simulink model "kfs_pr_2"  (R2019a)
settings: Solver=FixedStepAuto  StartTime=0.0  StopTime=30000  FixedStep=1  RelTol=1e-3
values from neighbouring files (symbols this model uses):
  mb = 10800    [params.m]
  min_paus = 100    [params.m]
  nurk = deg2rad(0)    [params.m]
  vx_0 = 0    [params.m]
  vy_0 = 0    [params.m]
  x_0 = 0    [params.m]
  x_OK = 100    [params.m]
  y_0 = 0    [params.m]
  y_OK = 0    [params.m]
libraries: simulink_extras x4, simulink x3, dspswit3 x2
settings Model: Creator=Kasutaja  LastModifiedBy=Kasutaja
settings DataIOCC: ReturnWorkspaceOutputs=off
settings DebuggingCC: ArithmeticOperatorsInVariantConditions=warning

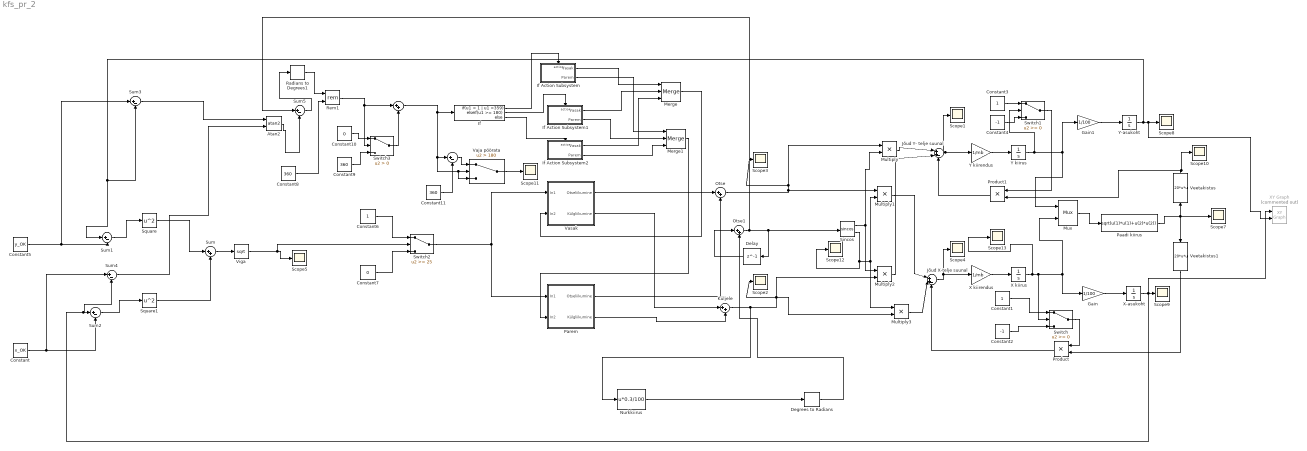
== system kfs_pr_2 ==
  " " : Sum  Inputs=|+-
  " " : Sum  Inputs=|++
  Atan2 : Trigonometry  Operator=atan2
  Constant : Constant  Value=x_OK
  Constant1 : Constant
  Constant10 : Constant  Value=0
  Constant11 : Constant  Value=360
  Constant2 : Constant  Value=-1
  Constant3 : Constant
  Constant4 : Constant  Value=-1
  Constant5 : Constant  Value=y_OK
  Constant6 : Constant
  Constant7 : Constant  Value=0
  Constant8 : Constant  Value=360
  Constant9 : Constant  Value=360
  Degrees to Radians : simulink_extras/Transformations/Degrees to Radians
  Delay : Delay  DelayLength=1  InitialCondition=nurk
  Gain : Gain  Gain=1/100
  Gain1 : Gain  Gain=1/100
  If : If  IfExpression=u1 < 1 | u1 >359  ElseIfExpressions=u1 >= 180
  If Action Subsystem : Subsystem  TreatAsAtomicUnit=on
  If Action Subsystem1 : Subsystem  TreatAsAtomicUnit=on
  If Action Subsystem2 : Subsystem  TreatAsAtomicUnit=on
  Jõud X-telje suunal : Sum  Inputs=|++-
  Jõud Y- telje suunal : Sum  Inputs=|++-
  Küljele : Sum  Inputs=|++
  Merge : Merge  Inputs=3
  Merge1 : Merge  Inputs=3
  Multiply{,1..3} (4 alike) : Product
  Mux : Mux  Inputs=2
      settings: DisplayOption=signals
  Nurkkiirus : Fcn  Expr=u*0.3/100
  Otse : Sum  Inputs=|++
  Otse1 : Sum  Inputs=|++
  Paadi kiirus : Fcn  Expr=sqrt(u(1)*u(1)+u(2)*u(2))
  Parem : Subsystem
  Product : Product
  Product1 : Product
  Radians to Degrees1 : simulink_extras/Transformations/Radians to Degrees
  Rem1 : Math  Operator=rem  SaturateOnIntegerOverflow=on
  Scope{1..5,7..13} (12 alike) : Scope
  Sincos : Trigonometry  Operator=sincos
  Square : Math  Operator=square  SaturateOnIntegerOverflow=on
  Square1 : Math  Operator=square  SaturateOnIntegerOverflow=on
  Sum : Sum  Inputs=|++
  Sum{1..5} (5 alike) : Sum  Inputs=|+-
  Switch : Switch
  Switch1 : Switch
  Switch2 : Switch  Threshold=25
  Switch3 : Switch  Criteria=u2 > Threshold
  Vaja pöörata : Switch  Criteria=u2 > Threshold  Threshold=180
  Vasak : Subsystem
  Veetakistus : Fcn  Expr=20*u*u
  Veetakistus1 : Fcn  Expr=20*u*u
  Viga : Sqrt  OutputSignalType=real  SaturateOnIntegerOverflow=on
  X kiirendus : Gain  Gain=1/mb
  X kiirus : Integrator  InitialCondition=vx_0
  X-asukoht : Integrator  InitialCondition=x_0
  XY Graph : simulink/Sinks/XY Graph  Commented=on  xmin=-20  xmax=20  ymin=-20  ymax=20  st=1
  Y kiirendus : Gain  Gain=1/mb
  Y kiirus : Integrator  InitialCondition=vy_0
  Y-asukoht : Integrator  InitialCondition=y_0
  wires:
  Vasak/1(Otseliikumine) -> Otse/1
  Otse/1 -> Multiply/1, Scope3/1, Multiply1/1
  Vasak/2(Külgliikumine) -> Küljele/1
  Küljele/1 -> Nurkkiirus/1, Multiply3/2, Multiply2/2, Scope2/1
  Sincos/1 -> Multiply2/1, Multiply/2
  Sincos/2 -> Scope12/1, Multiply1/2, Multiply3/1
  Multiply/1 -> Jõud Y- telje suunal/1
  Multiply2/1 -> Jõud Y- telje suunal/2
  Multiply3/1 -> Jõud X-telje suunal/2
  Multiply1/1 -> Jõud X-telje suunal/1
  Jõud Y- telje suunal/1 -> Scope1/1, Y kiirendus/1
  Jõud X-telje suunal/1 -> X kiirendus/1, Scope4/1
  X kiirendus/1 -> X kiirus/1
  Y kiirendus/1 -> Y kiirus/1
  Y kiirus/1 -> Switch1/2, Gain1/1, Mux/1
  X kiirus/1 -> Scope13/1, Switch/2, Mux/2, Gain/1
  Mux/1 -> Paadi kiirus/1
  Paadi kiirus/1 -> Veetakistus1/1, Veetakistus/1, Scope7/1
  Gain/1 -> X-asukoht/1
  Gain1/1 -> Y-asukoht/1
  Veetakistus/1 -> Product1/2, Scope10/1
  Veetakistus1/1 -> Product/2
  Constant1/1 -> Switch/1
  Constant2/1 -> Switch/3
  Switch/1 -> Product/1
  Product/1 -> Jõud X-telje suunal/3
  Constant3/1 -> Switch1/1
  Constant4/1 -> Switch1/3
  Switch1/1 -> Product1/1
  Product1/1 -> Jõud Y- telje suunal/3
  Nurkkiirus/1 -> Degrees to Radians/1
  Degrees to Radians/1 -> Otse1/2
  Delay/1 -> Otse1/1
  Square/1 -> Sum/1
  Square1/1 -> Sum/2
  Sum/1 -> Viga/1
  Viga/1 -> Switch2/2, Scope5/1
  Constant/1 -> Sum4/1, Sum2/2
  Constant5/1 -> Sum3/1, Sum1/2
  Y-asukoht/1 -> Sum3/2, Sum1/1, XY Graph/2, Scope8/1
  X-asukoht/1 -> XY Graph/1, Sum4/2, Sum2/1, Scope9/1
  Sum1/1 -> Square/1
  Sum2/1 -> Square1/1
  Constant6/1 -> Switch2/1
  Constant7/1 -> Switch2/3
  Switch2/1 -> Parem/1(In1), Vasak/1(In1)
  Sum4/1 -> Atan2/2
  Sum3/1 -> Atan2/1
  Atan2/1 -> Sum5/2
  Otse1/1 -> Sum5/1, Sincos/1, Delay/1
  Sum5/1 -> Radians to Degrees1/1
  Constant8/1 -> Rem1/2
  Rem1/1 -> " "/1, Switch3/2
  Radians to Degrees1/1 -> Rem1/1
  Constant10/1 -> Switch3/1
  Constant9/1 -> Switch3/3
  Switch3/1 -> " "/2
  If/1 -> If Action Subsystem/Action
  If/2 -> If Action Subsystem1/Action
  If/3 -> If Action Subsystem2/Action
  If Action Subsystem/1(Vasak) -> Merge/1
  If Action Subsystem1/1(Vasak) -> Merge/2
  If Action Subsystem2/1(Vasak) -> Merge/3
  If Action Subsystem2/2(Parem) -> Merge1/3
  If Action Subsystem1/2(Parem) -> Merge1/2
  If Action Subsystem/2(Parem) -> Merge1/1
  Merge/1 -> Vasak/2(In2)
  Merge1/1 -> Parem/2(In2)
  " "/1 -> Vaja pöörata/3, Vaja pöörata/2, " "/1, If/1
  Parem/1(Otseliikumine) -> Otse/2
  Parem/2(Külgliikumine) -> Küljele/2
  Vaja pöörata/1 -> Scope11/1
  Constant11/1 -> " "/2
  " "/1 -> Vaja pöörata/1

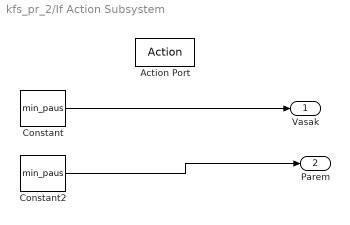
== system kfs_pr_2/If Action Subsystem ==
  Action Port : ActionPort  ActionPortLabel=if(u1 < 1 | u1 >359)
  Constant : Constant  Value=min_paus
  Constant2 : Constant  Value=min_paus
  Vasak : Outport
  Parem : Outport  Port=2
  wires:
  Constant/1 -> Vasak/1
  Constant2/1 -> Parem/1

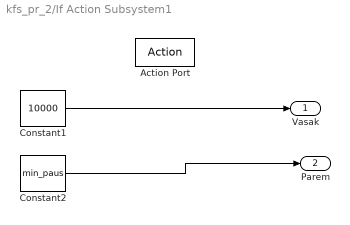
== system kfs_pr_2/If Action Subsystem1 ==
  Action Port : ActionPort  ActionPortLabel=elseif(u1 >= 180)
  Constant1 : Constant  Value=10000
  Constant2 : Constant  Value=min_paus
  Vasak : Outport
  Parem : Outport  Port=2
  wires:
  Constant1/1 -> Vasak/1
  Constant2/1 -> Parem/1

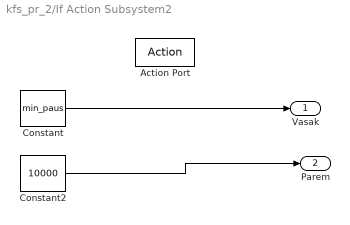
== system kfs_pr_2/If Action Subsystem2 ==
  Action Port : ActionPort  ActionPortLabel=else
  Constant : Constant  Value=min_paus
  Constant2 : Constant  Value=10000
  Vasak : Outport
  Parem : Outport  Port=2
  wires:
  Constant/1 -> Vasak/1
  Constant2/1 -> Parem/1

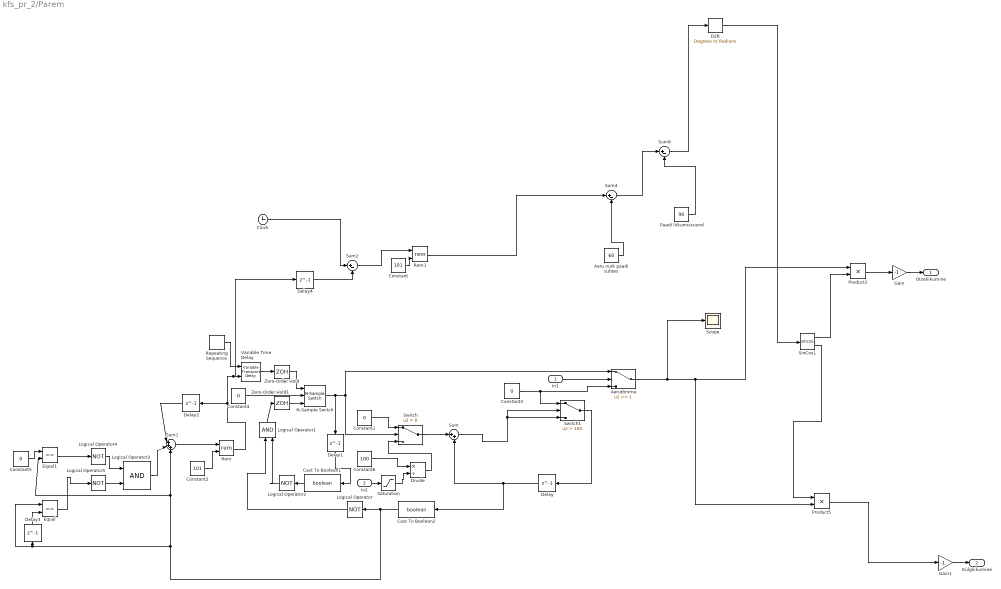
== system kfs_pr_2/Parem ==
  In1 : Inport
  In2 : Inport  Port=2
  Aeru nurk paadi suhtes : Constant  Value=60  SampleTime=1
  Aerutõmme : Switch  Threshold=1
  Cast To Boolean1 : DataTypeConversion  OutDataTypeStr=boolean
  Cast To Boolean2 : DataTypeConversion  OutDataTypeStr=boolean
  Clock : Clock
  Constant : Constant  Value=101
  Constant1 : Constant  Value=0
  Constant2 : Constant  Value=101  SampleTime=1
  Constant3 : Constant  Value=0
  Constant4 : Constant  Value=0  SampleTime=1
  Constant5 : Constant  Value=0
  Constant6 : Constant  Value=100  SampleTime=1
  D2R : simulink_extras/Transformations/Degrees to Radians
  Delay{,1..4} (5 alike) : Delay  DelayLength=1  InitialCondition=0
  Divide : Product  Inputs=*/
  Equal : RelationalOperator  Operator===  OutDataTypeStr=boolean  RndMeth=Simplest
  Equal1 : RelationalOperator  Operator===  OutDataTypeStr=boolean  RndMeth=Simplest
  Gain : Gain  Gain=-1
  Gain1 : Gain  Gain=-1
  Logical Operator{,2,4..5} (4 alike) : Logic  Operator=NOT  IconShape=distinctive  AllPortsSameDT=off  OutDataTypeStr=boolean
  Logical Operator1 : Logic  IconShape=distinctive  AllPortsSameDT=off  OutDataTypeStr=boolean
  Logical Operator3 : Logic  IconShape=distinctive  AllPortsSameDT=off  OutDataTypeStr=boolean
  N-Sample Switch : dspswit3/N-Sample Switch  N=101  reset=on  TriggerType=Non-zero sample  Ts=1
      settings: SourceProductName=DSP System Toolbox  SourceProductBaseCode=DS
  Paadi liikumissuund : Constant  Value=90  SampleTime=1
  Product2 : Product
  Product5 : Product
  Rem : Math  Operator=rem  SaturateOnIntegerOverflow=on
  Rem1 : Math  Operator=rem  SaturateOnIntegerOverflow=on
  Repeating Sequence : simulink/Sources/Repeating Sequence  rep_seq_t=|  rep_seq_y=|
      rep_seq_t=|
      | [0
      | 1
      | 2
      | 3
      | 4
      | 5
      | 6
      | 7
      | 8
      | 9
      | 10
      | 11
      | 12
      | 13
      | 14
      | 15
      | 16
      | 17
      | 18
      | 19
      | 20
      | 21
      | 22
      | 23
      | 24
      | 25
      | 26
      | 27
      | 28
      | 29
      | 30
      | 31
      | 32
      | 33
      | 34
      | 35
      | 36
      | 37
      | 38
      | 39
      | 40
      | 41
      | 42
      | 43
      | 44
      | 45
      | 46
      | 47
      | 48
      | 49
      | 50
      | 51
      | 52
      | 53
      | 54
      | 55
      | 56
      | 57
      | 58
      | 59
      | 60
      | 61
      | 62
      | 63
      | 64
      | 65
      | 66
      | 67
      | 68
      | 69
      | 70
      | 71
      | 72
      | 73
      | 74
      | 75
      | 76
      | 77
      | 78
      | 79
      | 80
      | 81
      | 82
      | 83
      | 84
      | 85
      | 86
      | 87
      | 88
      | 89
      | 90
      | 91
      | 92
      | 93
      | 94
      | 95
      | 96
      | 97
      | 98
      | 99
      | 100
      | 101  ]
      rep_seq_y=|
      | [1
      | 14
      | 28
      | 42
      | 56
      | 70
      | 84
      | 98
      | 112
      | 126
      | 167
      | 208
      | 249
      | 290
      | 331
      | 372
      | 413
      | 454
      | 495
      | 536
      | 551
      | 566
      | 581
      | 596
      | 611
      | 626
      | 641
      | 656
      | 671
      | 686
      | 697
      | 708
      | 719
      | 730
      | 741
      | 752
      | 763
      | 774
      | 785
      | 796
      | 801
      | 806
      | 811
      | 816
      | 821
      | 826
      | 831
      | 836
      | 841
      | 846
      | 841
      | 836
      | 831
      | 826
      | 821
      | 816
      | 811
      | 806
      | 801
      | 796
      | 785
      | 774
      | 763
      | 752
      | 741
      | 730
      | 719
      | 708
      | 697
      | 686
      | 646
      | 606
      | 566
      | 526
      | 486
      | 446
      | 406
      | 366
      | 326
      | 286
      | 279
      | 272
      | 265
      | 258
      | 251
      | 244
      | 237
      | 230
      | 223
      | 216
      | 198
      | 180
      | 162
      | 144
      | 126
      | 108
      | 90
      | 72
      | 54
      | 36
      | 18
      | -1  ]
  Saturation : Saturate  UpperLimit=10000  LowerLimit=min_paus
  Scope : Scope
  SinCos1 : Trigonometry  Operator=sincos
  Sum : Sum  Inputs=|++
  Sum1 : Sum  Inputs=|+++
  Sum2 : Sum  Inputs=|+-
  Sum4 : Sum  Inputs=|+-
  Sum9 : Sum  Inputs=|+-
  Switch : Switch  Criteria=u2 > Threshold
  Switch1 : Switch  Criteria=u2 > Threshold  Threshold=100
  Variable Time Delay : VariableTransportDelay  MaximumDelay=200  MaximumPoints=256  ZeroDelay=on
  Zero-Order Hold : ZeroOrderHold
  Zero-Order Hold1 : ZeroOrderHold
  Otseliikumine : Outport
  Külgliikumine : Outport  Port=2
  wires:
  Constant5/1 -> Equal1/1
  Logical Operator2/1 -> Logical Operator1/2
  Divide/1 -> Switch/3
  Logical Operator4/1 -> Logical Operator3/1
  N-Sample Switch/1 -> Aerutõmme/1, Switch/2, Delay1/1
  Sum/1 -> Switch1/3, Switch1/2
  Cast To Boolean1/1 -> Logical Operator2/1
  Equal1/1 -> Logical Operator4/1
  Constant3/1 -> Aerutõmme/3, Switch1/1
  Logical Operator/1 -> Logical Operator1/1
  Constant1/1 -> Switch/1
  Constant6/1 -> Divide/1
  Switch1/1 -> Delay/1
  In2/1 -> Saturation/1
  Cast To Boolean2/1 -> Sum1/3, Equal1/2, Delay3/1, Equal/1, Logical Operator/1
  Delay1/1 -> Cast To Boolean1/1
  Logical Operator1/1 -> Zero-Order Hold1/1
  Delay2/1 -> Sum1/1
  Delay/1 -> Cast To Boolean2/1, Sum/2
  Logical Operator5/1 -> Logical Operator3/2
  Constant4/1 -> N-Sample Switch/2
  Switch/1 -> Sum/1
  Zero-Order Hold/1 -> N-Sample Switch/1
  Variable Time Delay/1 -> Zero-Order Hold/1
  Delay3/1 -> Equal/2
  Logical Operator3/1 -> Sum1/2
  Equal/1 -> Logical Operator5/1
  Repeating Sequence/1 -> Variable Time Delay/1
  In1/1 -> Aerutõmme/2
  Clock/1 -> Sum2/1
  Sum2/1 -> Rem1/1
  Sum4/1 -> Sum9/1
  Aeru nurk paadi suhtes/1 -> Sum4/2
  Delay4/1 -> Sum2/2
  D2R/1 -> SinCos1/1
  SinCos1/1 -> Product2/2
  Aerutõmme/1 -> Scope/1, Product5/2, Product2/1
  Product5/1 -> Gain1/1
  SinCos1/2 -> Product5/1
  Product2/1 -> Gain/1
  Paadi liikumissuund/1 -> Sum9/2
  Sum9/1 -> D2R/1
  Gain1/1 -> Külgliikumine/1
  Gain/1 -> Otseliikumine/1
  Saturation/1 -> Divide/2
  Zero-Order Hold1/1 -> N-Sample Switch/3
  Sum1/1 -> Rem/1
  Rem/1 -> Delay2/1, Delay4/1, Variable Time Delay/2
  Constant2/1 -> Rem/2
  Rem1/1 -> Sum4/1
  Constant/1 -> Rem1/2

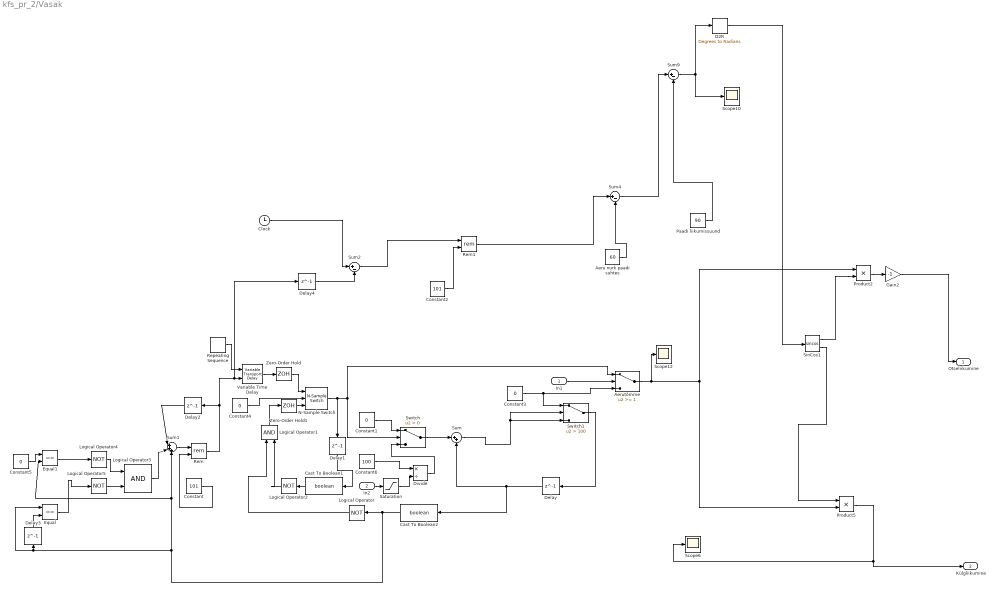
== system kfs_pr_2/Vasak ==
  In1 : Inport
  In2 : Inport  Port=2
  Aeru nurk paadi suhtes : Constant  Value=60  SampleTime=1
  Aerutõmme : Switch  Threshold=1
  Cast To Boolean1 : DataTypeConversion  OutDataTypeStr=boolean
  Cast To Boolean2 : DataTypeConversion  OutDataTypeStr=boolean
  Clock : Clock
  Constant : Constant  Value=101
  Constant{1,3..5} (4 alike) : Constant  Value=0
  Constant2 : Constant  Value=101
  Constant6 : Constant  Value=100  SampleTime=1
  D2R : simulink_extras/Transformations/Degrees to Radians
  Delay{,1..4} (5 alike) : Delay  DelayLength=1  InitialCondition=0
  Divide : Product  Inputs=*/
  Equal : RelationalOperator  Operator===  OutDataTypeStr=boolean  RndMeth=Simplest
  Equal1 : RelationalOperator  Operator===  OutDataTypeStr=boolean  RndMeth=Simplest
  Gain2 : Gain  Gain=-1
  Logical Operator{,2,4..5} (4 alike) : Logic  Operator=NOT  IconShape=distinctive  AllPortsSameDT=off  OutDataTypeStr=boolean
  Logical Operator1 : Logic  IconShape=distinctive  AllPortsSameDT=off  OutDataTypeStr=boolean
  Logical Operator3 : Logic  IconShape=distinctive  AllPortsSameDT=off  OutDataTypeStr=boolean
  N-Sample Switch : dspswit3/N-Sample Switch  N=101  reset=on  TriggerType=Non-zero sample  Ts=1
      settings: SourceProductName=DSP System Toolbox  SourceProductBaseCode=DS
  Paadi liikumissuund : Constant  Value=90  SampleTime=1
  Product2 : Product
  Product5 : Product
  Rem : Math  Operator=rem  SaturateOnIntegerOverflow=on
  Rem1 : Math  Operator=rem  SaturateOnIntegerOverflow=on
  Repeating Sequence : simulink/Sources/Repeating Sequence  rep_seq_t=|  rep_seq_y=|
      rep_seq_t=|
      | [0
      | 1
      | 2
      | 3
      | 4
      | 5
      | 6
      | 7
      | 8
      | 9
      | 10
      | 11
      | 12
      | 13
      | 14
      | 15
      | 16
      | 17
      | 18
      | 19
      | 20
      | 21
      | 22
      | 23
      | 24
      | 25
      | 26
      | 27
      | 28
      | 29
      | 30
      | 31
      | 32
      | 33
      | 34
      | 35
      | 36
      | 37
      | 38
      | 39
      | 40
      | 41
      | 42
      | 43
      | 44
      | 45
      | 46
      | 47
      | 48
      | 49
      | 50
      | 51
      | 52
      | 53
      | 54
      | 55
      | 56
      | 57
      | 58
      | 59
      | 60
      | 61
      | 62
      | 63
      | 64
      | 65
      | 66
      | 67
      | 68
      | 69
      | 70
      | 71
      | 72
      | 73
      | 74
      | 75
      | 76
      | 77
      | 78
      | 79
      | 80
      | 81
      | 82
      | 83
      | 84
      | 85
      | 86
      | 87
      | 88
      | 89
      | 90
      | 91
      | 92
      | 93
      | 94
      | 95
      | 96
      | 97
      | 98
      | 99
      | 100
      | 101  ]
      rep_seq_y=|
      | [1
      | 14
      | 28
      | 42
      | 56
      | 70
      | 84
      | 98
      | 112
      | 126
      | 167
      | 208
      | 249
      | 290
      | 331
      | 372
      | 413
      | 454
      | 495
      | 536
      | 551
      | 566
      | 581
      | 596
      | 611
      | 626
      | 641
      | 656
      | 671
      | 686
      | 697
      | 708
      | 719
      | 730
      | 741
      | 752
      | 763
      | 774
      | 785
      | 796
      | 801
      | 806
      | 811
      | 816
      | 821
      | 826
      | 831
      | 836
      | 841
      | 846
      | 841
      | 836
      | 831
      | 826
      | 821
      | 816
      | 811
      | 806
      | 801
      | 796
      | 785
      | 774
      | 763
      | 752
      | 741
      | 730
      | 719
      | 708
      | 697
      | 686
      | 646
      | 606
      | 566
      | 526
      | 486
      | 446
      | 406
      | 366
      | 326
      | 286
      | 279
      | 272
      | 265
      | 258
      | 251
      | 244
      | 237
      | 230
      | 223
      | 216
      | 198
      | 180
      | 162
      | 144
      | 126
      | 108
      | 90
      | 72
      | 54
      | 36
      | 18
      | -1  ]
  Saturation : Saturate  UpperLimit=100000  LowerLimit=min_paus
  Scope10 : Scope
  Scope12 : Scope
  Scope6 : Scope
  SinCos1 : Trigonometry  Operator=sincos
  Sum : Sum  Inputs=|++
  Sum1 : Sum  Inputs=|+++
  Sum2 : Sum  Inputs=|+-
  Sum4 : Sum  Inputs=|+-
  Sum9 : Sum  Inputs=|+-
  Switch : Switch  Criteria=u2 > Threshold
  Switch1 : Switch  Criteria=u2 > Threshold  Threshold=100
  Variable Time Delay : VariableTransportDelay  MaximumDelay=200  MaximumPoints=256  ZeroDelay=on
  Zero-Order Hold : ZeroOrderHold
  Zero-Order Hold1 : ZeroOrderHold
  Otseliikumine : Outport
  Külgliikumine : Outport  Port=2
  wires:
  Constant5/1 -> Equal1/1
  Logical Operator2/1 -> Logical Operator1/2
  Divide/1 -> Switch/3
  Logical Operator4/1 -> Logical Operator3/1
  N-Sample Switch/1 -> Aerutõmme/1, Switch/2, Delay1/1
  Sum/1 -> Switch1/3, Switch1/2
  Cast To Boolean1/1 -> Logical Operator2/1
  Equal1/1 -> Logical Operator4/1
  Constant3/1 -> Aerutõmme/3, Switch1/1
  Logical Operator/1 -> Logical Operator1/1
  Constant1/1 -> Switch/1
  Constant6/1 -> Divide/1
  Switch1/1 -> Delay/1
  In2/1 -> Saturation/1
  Cast To Boolean2/1 -> Sum1/3, Equal1/2, Delay3/1, Equal/1, Logical Operator/1
  Delay1/1 -> Cast To Boolean1/1
  Logical Operator1/1 -> Zero-Order Hold1/1
  Delay2/1 -> Sum1/1
  Delay/1 -> Cast To Boolean2/1, Sum/2
  Logical Operator5/1 -> Logical Operator3/2
  Constant4/1 -> N-Sample Switch/2
  Switch/1 -> Sum/1
  Zero-Order Hold/1 -> N-Sample Switch/1
  Variable Time Delay/1 -> Zero-Order Hold/1
  Delay3/1 -> Equal/2
  Logical Operator3/1 -> Sum1/2
  Equal/1 -> Logical Operator5/1
  Repeating Sequence/1 -> Variable Time Delay/1
  In1/1 -> Aerutõmme/2
  Clock/1 -> Sum2/1
  Sum4/1 -> Sum9/1
  Aeru nurk paadi suhtes/1 -> Sum4/2
  Delay4/1 -> Sum2/2
  D2R/1 -> SinCos1/1
  SinCos1/1 -> Product2/2
  Aerutõmme/1 -> Scope12/1, Product5/2, Product2/1
  SinCos1/2 -> Product5/1
  Product2/1 -> Gain2/1
  Paadi liikumissuund/1 -> Sum9/2
  Sum9/1 -> Scope10/1, D2R/1
  Gain2/1 -> Otseliikumine/1
  Saturation/1 -> Divide/2
  Zero-Order Hold1/1 -> N-Sample Switch/3
  Product5/1 -> Scope6/1, Külgliikumine/1
  Constant/1 -> Rem/2
  Sum1/1 -> Rem/1
  Rem/1 -> Delay2/1, Variable Time Delay/2, Delay4/1
  Sum2/1 -> Rem1/1
  Rem1/1 -> Sum4/1
  Constant2/1 -> Rem1/2
